simulink model "task_2s"  (R2021a)
settings: Solver=VariableStepAuto  StartTime=0  StopTime=100  RelTol=1e-3
values from neighbouring files (symbols this model uses):
  A_line = pi*D_line^2/4    (= 0.502654824574)    [task_2.m]    (also in task_3.m)
  A_p = pi*D_p^2/4    (= 0.441786466911)    [task_2.m]    (also in task_3.m)
  A_tank = pi*D_tank^2/4    (= 28.2743338823)    [task_2.m]    (also in task_3.m)
  beta_3 = 78*pi/180    (= 1.36135681656)    [task_2.m]    (also in task_3.m)
  Cd = 0.9    [task_2.m]    (also in task_3.m)
  D_line = 0.8    [task_2.m]    (also in task_3.m)
  D_p = 0.75    [task_2.m]    (also in task_3.m)
  D_w = 3.5    [task_2.m]    (also in task_3.m)
  g = 9.81    [task_2.m]    (also in task_3.m)
  h0 = 10    [task_2.m]    (also in task_3.m)
  h2 = 175    [task_2.m]    (also in task_3.m)
  h_tank_0 = 7.47    [task_2.m]    (also in task_3.m)
  K = 2e9    (= 2000000000)    [task_2.m]    (also in task_3.m)
  L_line = 5    [task_2.m]    (also in task_3.m)
  L_p = 220    [task_2.m]    (also in task_3.m)
  lambda = 5e-3    (= 0.005)    [task_2.m]    (also in task_3.m)
  lambda_p = 1e-4    (= 0.0001)    [task_2.m]    (also in task_3.m)
  omega_t = 15    [task_2.m]    (also in task_3.m)
  p_amb = 1e5    (= 100000)    [task_2.m]    (also in task_3.m)
  psi = 0.97    [task_2.m]    (also in task_3.m)
  rho = 1000    [task_2.m]    (also in task_3.m)
  Rv = (Av0/pi)^(1/2)    (= 0.398942280401)    [task_2.m]    (also in task_3.m)
  V_c = 0.27    [task_2.m]    (also in task_3.m)
  V_p = A_p*L_p    (= 97.1930227204)    [task_2.m]    (also in task_3.m)
  x_v = 0.5    [task_2.m]    (also in task_3.m)
undefined symbols (not defined in the file or in its folder): magnitude
settings Model: Creator=Jihai  LastModifiedBy=nakah
settings SolverCC: AlgebraicLoopSolver=TrustRegion
settings OptimizationCC: BlockReduction=off  DefaultParameterBehavior=Inlined  BufferReuse=off
settings DebuggingCC: SFMachineParentedDataDiag=warning

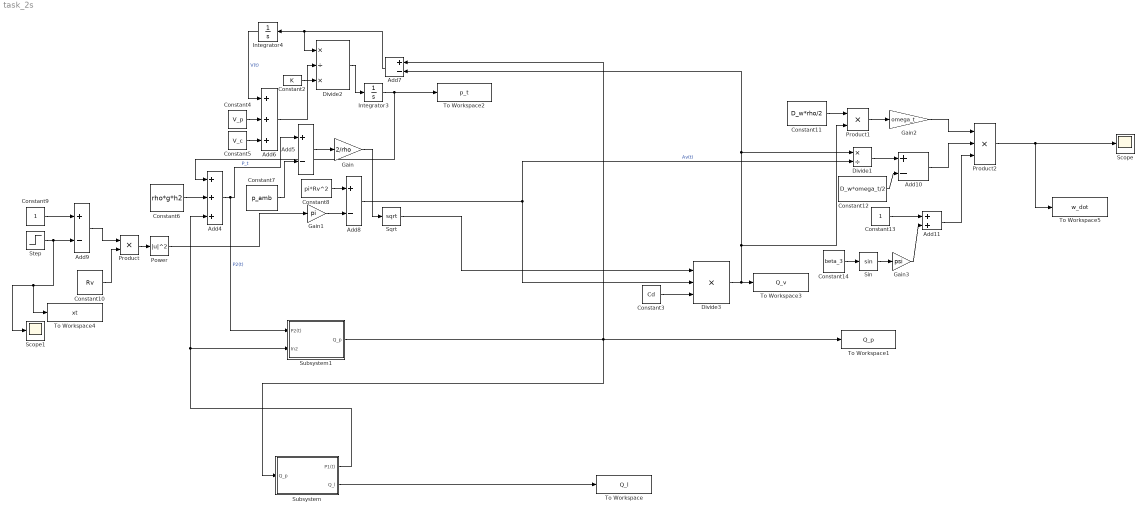
== system task_2s ==
  Add{5,7..10} (5 alike) : Sum  Inputs=+-
  Add11 : Sum
  Add4 : Sum  Inputs=+++
  Add6 : Sum  Inputs=+++
  Constant10 : Constant  Value=Rv
  Constant11 : Constant  Value=D_w*rho/2
  Constant12 : Constant  Value=D_w*omega_t/2
  Constant13 : Constant
  Constant14 : Constant  Value=beta_3
  Constant2 : Constant  Value=K
  Constant3 : Constant  Value=Cd
  Constant4 : Constant  Value=V_p
  Constant5 : Constant  Value=V_c
  Constant6 : Constant  Value=rho*g*h2
  Constant7 : Constant  Value=p_amb
  Constant8 : Constant  Value=pi*Rv^2
  Constant9 : Constant
  Divide1 : Product  Inputs=*/
  Divide2 : Product  Inputs=*/*
  Divide3 : Product  Inputs=***
  Gain : Gain  Gain=2/rho
  Gain1 : Gain  Gain=pi
  Gain2 : Gain  Gain=omega_t
  Gain3 : Gain  Gain=psi
  Integrator3 : Integrator
  Integrator4 : Integrator
  Power : Math  Operator=magnitude^2  SaturateOnIntegerOverflow=on
  Product : Product
  Product1 : Product
  Product2 : Product  Inputs=3
  Scope : Scope
  Scope1 : Scope
  Sin : Trigonometry
  Sqrt : Sqrt  SaturateOnIntegerOverflow=on
  Step : Step  Time=50  Before=x_v  After=0.6  SampleTime=0
  Subsystem : Subsystem
  Subsystem1 : Subsystem
  To Workspace : ToWorkspace  VariableName=Q_l  SampleTime=-1
  To Workspace1 : ToWorkspace  VariableName=Q_p  SampleTime=-1
  To Workspace2 : ToWorkspace  VariableName=p_t  SampleTime=-1
  To Workspace3 : ToWorkspace  VariableName=Q_v  SampleTime=-1
  To Workspace4 : ToWorkspace  VariableName=xt  SaveFormat=Timeseries  SampleTime=-1
  To Workspace5 : ToWorkspace  VariableName=w_dot  SaveFormat=Timeseries  SampleTime=-1
  wires:
  Add6/1 -> Divide2/2
  Divide2/1 -> Integrator3/1
  Constant2/1 -> Divide2/3
  Integrator4/1 -> Add6/1  "V(t)"
  Constant4/1 -> Add6/2
  Constant5/1 -> Add6/3
  Add7/1 -> Divide2/1, Integrator4/1
  Divide3/1 -> Divide1/1, Add7/2, Product1/2, To Workspace3/1
  Constant3/1 -> Divide3/3
  Constant6/1 -> Add4/2
  Integrator3/1 -> To Workspace2/1, Add4/1  "P_t"
  Add4/1 -> Subsystem1/1(P2(t)), Add5/1  "P2(t)"
  Constant7/1 -> Add5/2
  Add5/1 -> Gain/1
  Gain/1 -> Sqrt/1
  Constant8/1 -> Add8/1
  Constant9/1 -> Add9/1
  Constant10/1 -> Product/2
  Add9/1 -> Product/1
  Product/1 -> Power/1
  Power/1 -> Gain1/1
  Gain1/1 -> Add8/2
  Add8/1 -> Divide1/2, Divide3/2  "Av(t)"
  Constant11/1 -> Product1/1
  Product1/1 -> Gain2/1
  Divide1/1 -> Add10/1
  Constant12/1 -> Add10/2
  Gain2/1 -> Product2/1
  Add10/1 -> Product2/2
  Constant13/1 -> Add11/1
  Constant14/1 -> Sin/1
  Sin/1 -> Gain3/1
  Gain3/1 -> Add11/2
  Add11/1 -> Product2/3
  Product2/1 -> To Workspace5/1, Scope/1
  Subsystem/1(P1(t)) -> Add4/3, Subsystem1/2(In2)
  Subsystem/2(Q_l) -> To Workspace/1
  Subsystem1/1(Q_p) -> Subsystem/1(Q_p), To Workspace1/1, Add7/1
  Sqrt/1 -> Divide3/1
  Step/1 -> To Workspace4/1, Scope1/1, Add9/2

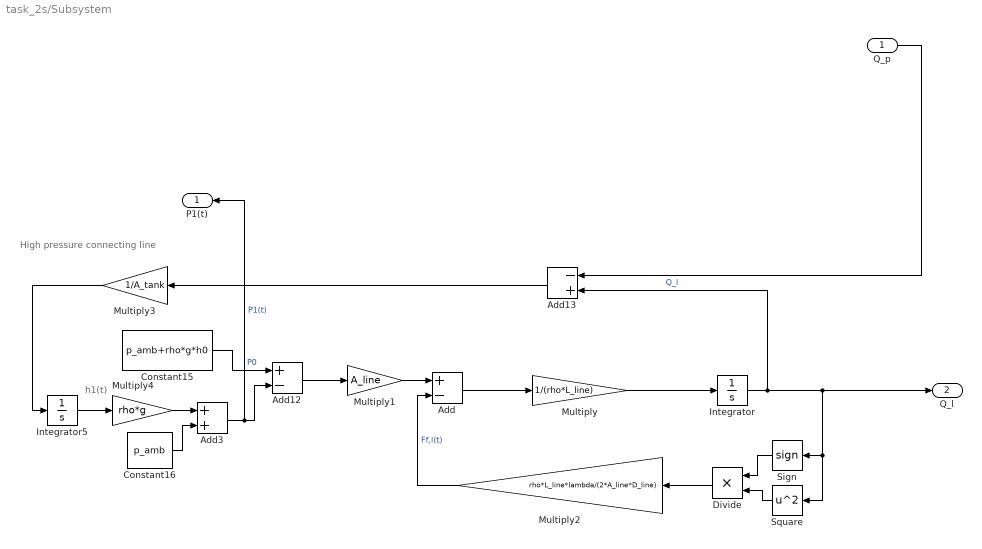
== system task_2s/Subsystem ==
  note: High pressure connecting line
  note: h1(t)
  Q_p : Inport
  Add : Sum  Inputs=+-
  Add12 : Sum  Inputs=+-
  Add13 : Sum  Inputs=-+
  Add3 : Sum
  Constant15 : Constant  Value=p_amb+rho*g*h0
  Constant16 : Constant  Value=p_amb
  Divide : Product  Inputs=**
  Integrator : Integrator  InitialCondition=20
  Integrator5 : Integrator  InitialCondition=h_tank_0
  Multiply : Gain  Gain=1/(rho*L_line)
  Multiply1 : Gain  Gain=A_line
  Multiply2 : Gain  Gain=rho*L_line*lambda/(2*A_line*D_line)
  Multiply3 : Gain  Gain=1/A_tank
  Multiply4 : Gain  Gain=rho*g
  Sign : Signum
  Square : Math  Operator=square  SaturateOnIntegerOverflow=on
  P1(t) : Outport
  Q_l : Outport  Port=2
  wires:
  Integrator/1 -> Q_l/1, Sign/1, Square/1, Add13/2  "Q_l"
  Constant16/1 -> Add3/2
  Multiply4/1 -> Add3/1
  Q_p/1 -> Add13/1
  Multiply/1 -> Integrator/1
  Add/1 -> Multiply/1
  Constant15/1 -> Add12/1  "P0"
  Divide/1 -> Multiply2/1
  Add13/1 -> Multiply3/1
  Add12/1 -> Multiply1/1
  Multiply3/1 -> Integrator5/1
  Integrator5/1 -> Multiply4/1
  Multiply1/1 -> Add/1
  Add3/1 -> Add12/2, P1(t)/1  "P1(t)"
  Sign/1 -> Divide/1
  Square/1 -> Divide/2
  Multiply2/1 -> Add/2  "Ff,l(t)"

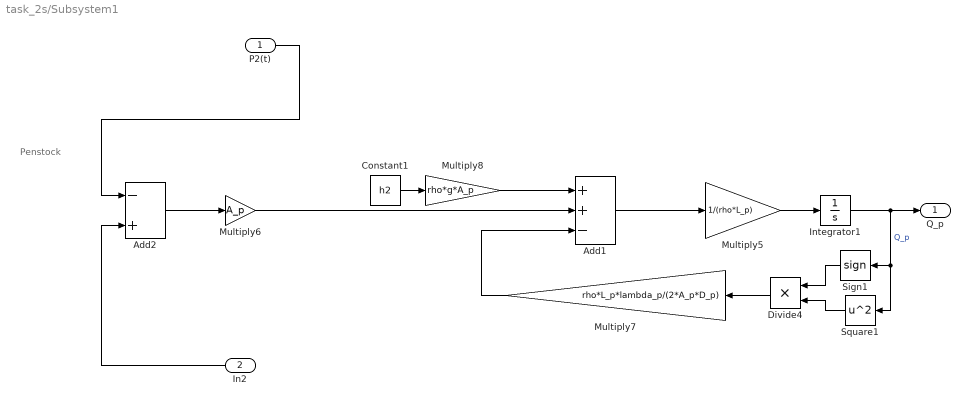
== system task_2s/Subsystem1 ==
  note: Penstock
  P2(t) : Inport
  In2 : Inport  Port=2
  Add1 : Sum  Inputs=++-
  Add2 : Sum  Inputs=-+
  Constant1 : Constant  Value=h2
  Divide4 : Product  Inputs=**
  Integrator1 : Integrator  InitialCondition=20
  Multiply5 : Gain  Gain=1/(rho*L_p)
  Multiply6 : Gain  Gain=A_p
  Multiply7 : Gain  Gain=rho*L_p*lambda_p/(2*A_p*D_p)
  Multiply8 : Gain  Gain=rho*g*A_p
  Sign1 : Signum
  Square1 : Math  Operator=square  SaturateOnIntegerOverflow=on
  Q_p : Outport
  wires:
  Add2/1 -> Multiply6/1
  In2/1 -> Add2/2
  Integrator1/1 -> Q_p/1, Square1/1, Sign1/1  "Q_p"
  Multiply7/1 -> Add1/3
  Divide4/1 -> Multiply7/1
  Add1/1 -> Multiply5/1
  Square1/1 -> Divide4/2
  Multiply5/1 -> Integrator1/1
  Sign1/1 -> Divide4/1
  Multiply8/1 -> Add1/1
  Multiply6/1 -> Add1/2
  Constant1/1 -> Multiply8/1
  P2(t)/1 -> Add2/1
